simulink library "csci_fsw_lib"  (R2015b)
settings: Solver=ode45  StartTime=0.0  StopTime=10.0  RelTol=1e-3
libraries: util_info_lib x1, csc_act_actuator_manager_lib x1, csc_cmp_command_mode_process_lib x1, csc_cnt_attitude_control_lib x1, csc_estimation_lib x1, csc_gdn_guidance_lib x1, csc_hio_hardware_io_lib x1, csc_lc_limit_check_lib x1, csc_sc_wsim_stored_command_lib x1, csu_cfe_cfe_time_lib x1, csu_tlm_telemetry_lib x1
settings Model: Creator=jkaidy  LastModifiedBy=jimkaidy
settings DataIOCC: SaveFormat=Array  SignalLoggingSaveFormat=ModelDataLogs
settings OptimizationCC: ExpressionDepthLimit=2147483647
settings DebuggingCC: UnderspecifiedInitializationDetection=Classic  MergeDetectMultiDrivingBlocksExec=none  SolverPrmCheckMsg=warning  FcnCallInpInsideContextMsg=EnableAllAsWarning  StateNameClashWarn=warning
settings HardwareCC: ProdBitPerPointer=32  ProdLargestAtomicFloat=None  ProdIntDivRoundTo=Undefined  ProdEndianess=Unspecified  ProdWordSize=32  ProdHWDeviceType=32-bit Generic
settings GRTTargetCC: GeneratePreprocessorConditionals=Disable all
settings ConfigComp: CovModelRefEnable=Off  CovSFcnEnable=off

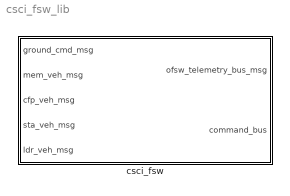
== system csci_fsw_lib ==
  csci_fsw : Subsystem

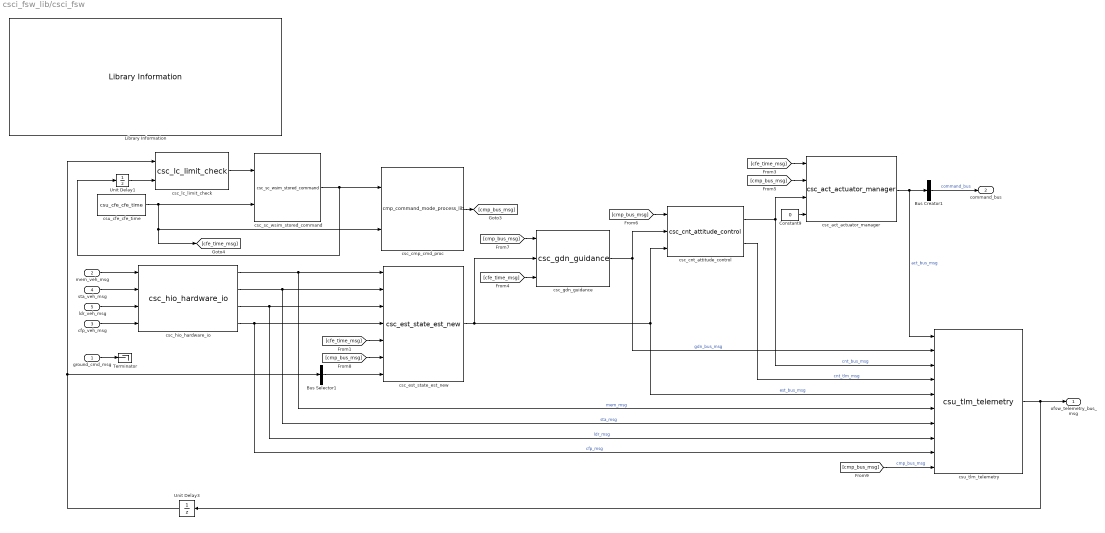
== system csci_fsw_lib/csci_fsw ==
  ground_cmd_msg : Inport
  mem_veh_msg : Inport  Port=2
  cfp_veh_msg : Inport  Port=3
  sta_veh_msg : Inport  Port=4
  ldr_veh_msg : Inport  Port=5
  Bus Creator1 : BusCreator  Inputs=1
  Bus Selector1 : BusSelector  OutputSignals=act_bus_msg  OutputAsBus=on
  Constant9 : Constant  Value=0  OutDataTypeStr=uint32
  Library Information : util_info_lib/Library Information  owner='NONE'
  Terminator : Terminator
  Unit Delay1 : UnitDelay  SampleTime=-1
  Unit Delay3 : UnitDelay  SampleTime=-1
  csc_act_actuator_manager : csc_act_actuator_manager_lib/csc_act_actuator_manager  Tag=OFSW; MDL_TICK=CNT_BUS_MSG
  csc_cmp_cmd_proc : csc_cmp_command_mode_process_lib/cmp_command_mode_process_lib  Tag=OFSW
  csc_cnt_attitude_control : csc_cnt_attitude_control_lib/csc_cnt_attitude_control  Tag=OFSW; MDL_TICK=GDN_BUS_MSG
  csc_est_state_est_new : csc_estimation_lib/csc_est_state_est_new  Tag=OFSW; MDL_TICK=CMP_BUS_MSG
  csc_gdn_guidance : csc_gdn_guidance_lib/csc_gdn_guidance  Tag=OFSW; MDL_TICK=EST_BUS_MSG
  csc_hio_hardware_io : csc_hio_hardware_io_lib/csc_hio_hardware_io
  csc_lc_limit_check : csc_lc_limit_check_lib/csc_lc_limit_check
  csc_sc_wsim_stored_command : csc_sc_wsim_stored_command_lib/csc_sc_wsim_stored_command
  csu_cfe_cfe_time : csu_cfe_cfe_time_lib/csu_cfe_cfe_time  sch_dt=fsw_dt
  csu_tlm_telemetry : csu_tlm_telemetry_lib/csu_tlm_telemetry  num_inputs=10  output_bus_name=ofsw_telemetry_bus_msg
  ofsw_telemetry_bus_msg : Outport
  command_bus : Outport  Port=2
  wires:
  csc_hio_hardware_io/1 -> csu_tlm_telemetry/6, csc_est_state_est_new/1  "mem_msg"
  mem_veh_msg/1 -> csc_hio_hardware_io/1
  Constant9/1 -> csc_act_actuator_manager/4
  csc_act_actuator_manager/1 -> Bus Creator1/1, csu_tlm_telemetry/1  "act_bus_msg"
  [cmp_bus_msg] -> csc_act_actuator_manager/2
  [cfe_time_msg] -> csc_act_actuator_manager/1
  Bus Selector1/1 -> csc_est_state_est_new/7
  [cmp_bus_msg] -> csc_est_state_est_new/6
  csc_sc_wsim_stored_command/1 -> csc_cmp_cmd_proc/1, Unit Delay1/1
  csc_est_state_est_new/1 -> csc_cnt_attitude_control/3, csu_tlm_telemetry/5, csc_gdn_guidance/2  "est_bus_msg"
  csc_cnt_attitude_control/1 -> csu_tlm_telemetry/3, csc_act_actuator_manager/3  "cnt_bus_msg"
  ground_cmd_msg/1 -> Terminator/1
  csc_gdn_guidance/1 -> csu_tlm_telemetry/2, csc_cnt_attitude_control/2  "gdn_bus_msg"
  csu_tlm_telemetry/1 -> Unit Delay3/1, ofsw_telemetry_bus_msg/1
  Bus Creator1/1 -> command_bus/1  "command_bus"
  [cfe_time_msg] -> csc_gdn_guidance/3
  csu_cfe_cfe_time/1 -> csc_sc_wsim_stored_command/2, csc_cmp_cmd_proc/2, [cfe_time_msg]
  csc_cmp_cmd_proc/1 -> [cmp_bus_msg]
  [cfe_time_msg] -> csc_est_state_est_new/5
  [cmp_bus_msg] -> csc_cnt_attitude_control/1
  [cmp_bus_msg] -> csc_gdn_guidance/1
  csc_cnt_attitude_control/2 -> csu_tlm_telemetry/4  "cnt_tlm_msg"
  sta_veh_msg/1 -> csc_hio_hardware_io/2
  ldr_veh_msg/1 -> csc_hio_hardware_io/3
  cfp_veh_msg/1 -> csc_hio_hardware_io/4
  csc_hio_hardware_io/2 -> csu_tlm_telemetry/7, csc_est_state_est_new/2  "sta_msg"
  csc_hio_hardware_io/3 -> csu_tlm_telemetry/8, csc_est_state_est_new/3  "ldr_msg"
  csc_hio_hardware_io/4 -> csu_tlm_telemetry/9, csc_est_state_est_new/4  "cfp_msg"
  [cmp_bus_msg] -> csu_tlm_telemetry/10  "cmp_bus_msg"
  csc_lc_limit_check/1 -> csc_sc_wsim_stored_command/1
  Unit Delay3/1 -> Bus Selector1/1, csc_lc_limit_check/1
  Unit Delay1/1 -> csc_lc_limit_check/2
